simulink model "test_case_2"  (R2017b)
settings: Solver=VariableStepAuto  StartTime=0.0  StopTime=10.0  RelTol=1e-3
libraries: DigitalControlLib2 x4, realtime_pacer_lib x1
settings Model: Creator=alexandersoussan  LastModifiedBy=alexandersoussan

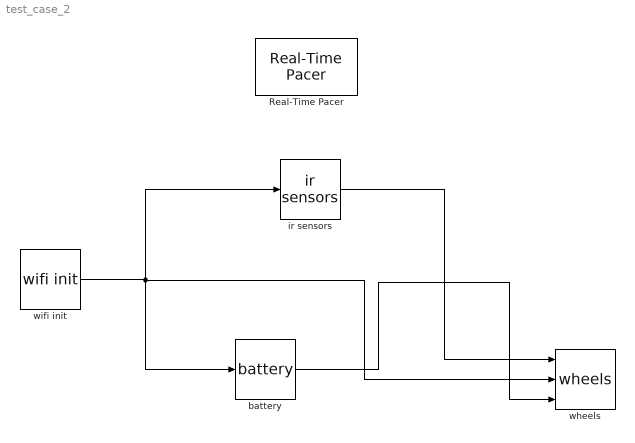
== system test_case_2 ==
  Real-Time Pacer : realtime_pacer_lib/Real-Time Pacer  simTimePerRealTime=1
  battery : DigitalControlLib2/battery
  ir sensors : DigitalControlLib2/ir sensors
  wheels : DigitalControlLib2/wheels
  wifi init : DigitalControlLib2/wifi init
  wires:
  battery/1 -> wheels/3
  ir sensors/1 -> wheels/1
  wifi init/1 -> ir sensors/1, wheels/2, battery/1
